simulink library "Pressure_Drop_Fix"  (R2016b)
settings: Solver=ode45  StartTime=0.0  StopTime=10.0  RelTol=1e-3  EnableMultiTasking=on
undefined symbols (not defined in the file): DPConstant, DPLinear, DPQuadratic, Pressure
libraries: carnot x1
settings Model: Creator=drhf  LastModifiedBy=drhf
settings DataIOCC: LimitDataPoints=on  SaveFormat=Array  SignalLoggingSaveFormat=ModelDataLogs
settings OptimizationCC: ExpressionDepthLimit=2147483647  LifeSpan=inf
settings DebuggingCC: UnderspecifiedInitializationDetection=Classic  MergeDetectMultiDrivingBlocksExec=none  SolverPrmCheckMsg=warning  FcnCallInpInsideContextMsg=warning  StateNameClashWarn=warning  SFUnexpectedBacktrackingDiag=warning  SFNoUnconditionalDefaultTransitionDiag=warning  SFExecutionAtInitializationDiag=none
settings HardwareCC: ProdBitPerPointer=32  ProdBitPerSizeT=32  ProdBitPerPtrDiffT=32  ProdLargestAtomicFloat=None  ProdIntDivRoundTo=Undefined  ProdEndianess=Unspecified  ProdWordSize=32  ProdHWDeviceType=32-bit Generic
settings ModelReferenceCC: PropagateSignalLabelsOutOfModel=off
settings GRTTargetCC: TargetLangStandard=C89/C90 (ANSI)  GeneratePreprocessorConditionals=Disable all  CombineOutputUpdateFcns=off  GRTInterface=on
settings ConfigComp: CovMetricSettings=dw  CovHtmlReporting=on  CovSaveCumulativeToWorkspaceVar=on  CovSaveSingleToWorkspaceVar=on  CovExternalEMLEnable=off

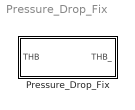
== system Pressure_Drop_Fix ==
  Pressure_Drop_Fix : Subsystem  mask(fixed pressure drop){con=101, lin=202, qua=303}
      mask prompts: con "c : constant (static) pressure drop in Pa"; lin "l : linear pressure drop Pa/(kg/s)"; qua "q : quadratic pressure drop Pa/(kg/s)²"
      mask help:
      | Constant parameters for pressure drop in a flow.
      | dp = c + l*mdot + q*mdot²
      | Calculation is done for ID > 10000 (dp = f(l, q), c is neglected) and ID > 20000 (dp = f(c,l,q)).
      | Applied directly to the THB bus.
      mask Help: web(fullfile(path_carnot('help'),'Pressure_Drop_Fix.html'),'-helpbrowser')

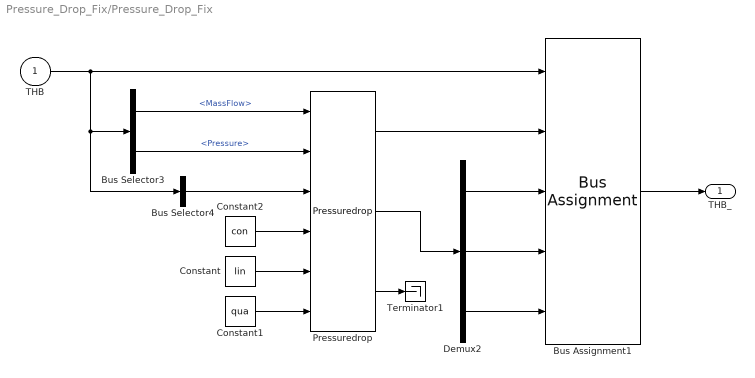
== system Pressure_Drop_Fix/Pressure_Drop_Fix ==
  THB : Inport
  Bus Assignment1 : BusAssignment  AssignedSignals=Pressure,DPConstant,DPLinear,DPQuadratic
  Bus Selector3 : BusSelector  OutputSignals=MassFlow,Pressure
  Bus Selector4 : BusSelector  OutputSignals=DPConstant,DPLinear,DPQuadratic  OutputAsBus=on
  Constant : Constant  Value=lin
  Constant1 : Constant  Value=qua
  Constant2 : Constant  Value=con
  Demux2 : Demux  Outputs=3
  Pressuredrop : carnot/Basic/Pressure_Drop/Pressuredrop
  Terminator1 : Terminator
  THB_ : Outport
  wires:
  Pressuredrop/2 -> Demux2/1
  Pressuredrop/1 -> Bus Assignment1/2
  Constant1/1 -> Pressuredrop/6
  Constant/1 -> Pressuredrop/5
  Constant2/1 -> Pressuredrop/4
  Bus Selector4/1 -> Pressuredrop/3
  Bus Selector3/2 -> Pressuredrop/2  "<Pressure>"
  Bus Selector3/1 -> Pressuredrop/1  "<MassFlow>"
  Demux2/3 -> Bus Assignment1/5
  Demux2/2 -> Bus Assignment1/4
  Demux2/1 -> Bus Assignment1/3
  Bus Assignment1/1 -> THB_/1
  THB/1 -> Bus Selector3/1, Bus Selector4/1, Bus Assignment1/1
  Pressuredrop/3 -> Terminator1/1
